simulink model "switched_load_R2021a"  (R2021a)
settings: Solver=VariableStepAuto  StartTime=0.0  StopTime=3  RelTol=1e-3
libraries: spsDiodeLib x15, spsSeriesRLCBranchLib x13, spsIGBTDiodeLib x12, spsVoltageMeasurementLib x6, spsCurrentMeasurementLib x6, simulink x2, spsIGBTLib x2, spsThreePhaseVIMeasurementLib x1, spsThreePhaseSourceLib x1, spsGroundLib x1, spspowerguiLib x1
settings Model: Creator=amogh  LastModifiedBy=amogh
settings DebuggingCC: UnconnectedInputMsg=none  UnconnectedOutputMsg=none  UnconnectedLineMsg=none
settings ModelReferenceCC: EnableRefExpFcnMdlSchedulingChecks=off
settings RTWCC: Description=Generic Real-Time Target  GPUComputeCapability=5.0  DLArmComputeVersion=20.02.1

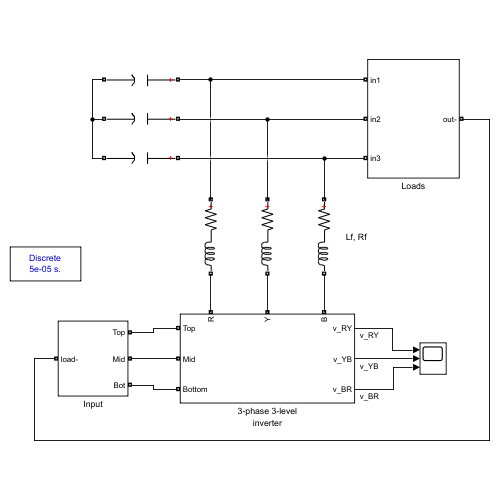
[thumbnail: Simulink's stored preview of the top-level diagram]
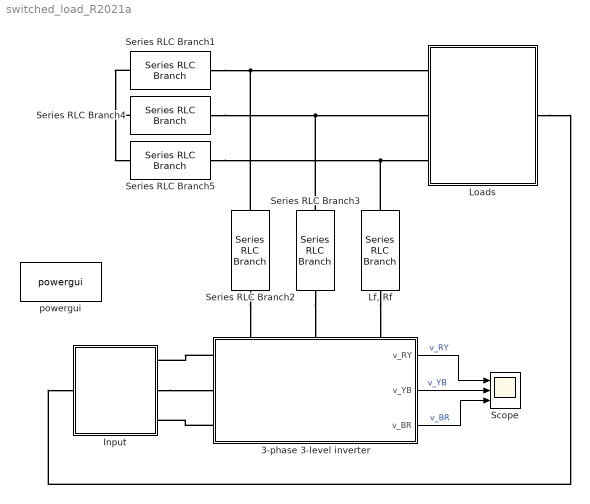
== system switched_load_R2021a ==
  3-phase 3-level inverter : Subsystem
      settings: PortSchema="{\"entries\":[{\"content\":{\"sides\":[{\"content\":{\"connectorIds\":[\"LConn1\",\"LConn2\",\"LConn3\"]},\"type\":\"ConnectorPlacement.EquallySpacedRectSide\",\"uuid\":\"13d4cf2c-4c1e-42a3-9432-c4e4ea2c8c55\"},{\"content\":{\"connectorIds\":[\"Out1\",\"Out2\",\"Out3\"],\"side\":\"RIGHT\"},\"type\":\"ConnectorPlacement.EquallySpacedRectSide\",\"uuid\":\"789192d8-f493-444e-b6ae-5a6372a819a0\"},{\"content\":{\"connectorIds\":[\"LConn4\",\"LConn5\",\"LConn6\"],\"side\":\"TOP\"},\"type\":\"ConnectorPlacement.EquallySpacedRectSide\",\"uuid\":\"d4a8605d-32e8-489f-b368-c8e22b15ad13\"}]},\"type\":\"ConnectorPlacement.EquallySpacedConnector\",\"uuid\":\"3af644a1-665b-410e-abe8-e1731342a0b4\"}],\"packageUris\":[\"http://schema.mathworks.com/mf0/Connector/R2020b\"],\"version\":\"1.0\"}"
  Input : Subsystem
  "Lf, Rf" : spsSeriesRLCBranchLib/Series RLC Branch  LConnTagsString=__new0  RConnTagsString=__new0  BranchType=RL  Resistance=0.01  Inductance=20e-3  SetiL0=off  InitialCurrent=0  Capacitance=1e-6  Setx0=off  InitialVoltage=0  Measurements=None
  Loads : Subsystem
  Scope : Scope  NumInputPorts=3
  Series RLC Branch1 : spsSeriesRLCBranchLib/Series RLC Branch  LConnTagsString=__new0  RConnTagsString=__new0  BranchType=C  Resistance=1  Inductance=20e-3  SetiL0=off  InitialCurrent=0  Capacitance=40e-6  Setx0=off  InitialVoltage=0  Measurements=None
  Series RLC Branch2 : spsSeriesRLCBranchLib/Series RLC Branch  LConnTagsString=__new0  RConnTagsString=__new0  BranchType=RL  Resistance=0.01  Inductance=20e-3  SetiL0=off  InitialCurrent=0  Capacitance=1e-6  Setx0=off  InitialVoltage=0  Measurements=None
  Series RLC Branch3 : spsSeriesRLCBranchLib/Series RLC Branch  LConnTagsString=__new0  RConnTagsString=__new0  BranchType=RL  Resistance=0.01  Inductance=20e-3  SetiL0=off  InitialCurrent=0  Capacitance=1e-6  Setx0=off  InitialVoltage=0  Measurements=None
  Series RLC Branch4 : spsSeriesRLCBranchLib/Series RLC Branch  LConnTagsString=__new0  RConnTagsString=__new0  BranchType=C  Resistance=1  Inductance=20e-3  SetiL0=off  InitialCurrent=0  Capacitance=40e-6  Setx0=off  InitialVoltage=0  Measurements=None
  Series RLC Branch5 : spsSeriesRLCBranchLib/Series RLC Branch  LConnTagsString=__new0  RConnTagsString=__new0  BranchType=C  Resistance=1  Inductance=20e-3  SetiL0=off  InitialCurrent=0  Capacitance=40e-6  Setx0=off  InitialVoltage=0  Measurements=None
  powergui : spspowerguiLib/powergui  Priority=1  SimulationMode=Discrete  SampleTime=50e-6  frequency=60  Iterations=50  frequencyindice=0  Pbase=100e6  ErrMax=1e-4  UnitsV=kV  UnitsW=MW  buscounter=0  FunctionMessages=off  echomessages=off  EnableUseOfTLC=off  CurrentSourceSwitches=off  DisableSnubberDevices=off  DisableRonSwitches=off  DisableVfSwitches=off  DisplayEquations=off  AutomaticDiscreteSolvers=off  SolverType=Tustin/Backward Euler (TBE)  Interpol=off  ExternalGateDelay=off  methode=off  Ts=100  x0status=blocks  SPID=on  SwTol=0  HookPort=off  NonlinearTolerance=1e-4  nMaxIteration=100  ContinueOnMaxIteration=off  RestoreLinks=warning  ResistiveCurrentMeasurement=off  Frange=[0:2:500]  Ylog=off  Xlog=on  ShowGrid=off  save=off  variable=ZData  structure=0  ZoomFFT=off  StartTime=0.0  cycles=1  DisplayStyle=1  fundamental=60  FreqAxis=off  MaxFrequency=1000  frequencyindicesteady=1  RmsSteady=1  display=off
  wires:
  3-phase 3-level inverter/3(v_BR) -> Scope/3  "v_BR"
  3-phase 3-level inverter/2(v_YB) -> Scope/2  "v_YB"
  3-phase 3-level inverter/1(v_RY) -> Scope/1  "v_RY"
  connections:
  Series RLC Branch1/LConn1 -- Loads/LConn1 -- Series RLC Branch2/LConn1
  Series RLC Branch5/LConn1 -- Loads/LConn3 -- "Lf, Rf"/LConn1
  Series RLC Branch4/RConn1 -- Series RLC Branch5/RConn1 -- Series RLC Branch1/RConn1
  Series RLC Branch4/LConn1 -- Loads/LConn2 -- Series RLC Branch3/LConn1
  3-phase 3-level inverter/LConn3 -- Input/RConn3
  Input/RConn2 -- 3-phase 3-level inverter/LConn2
  3-phase 3-level inverter/LConn1 -- Input/RConn1
  Series RLC Branch2/RConn1 -- 3-phase 3-level inverter/LConn4
  Series RLC Branch3/RConn1 -- 3-phase 3-level inverter/LConn5
  "Lf, Rf"/RConn1 -- 3-phase 3-level inverter/LConn6
  Loads/RConn1 -- Input/LConn1

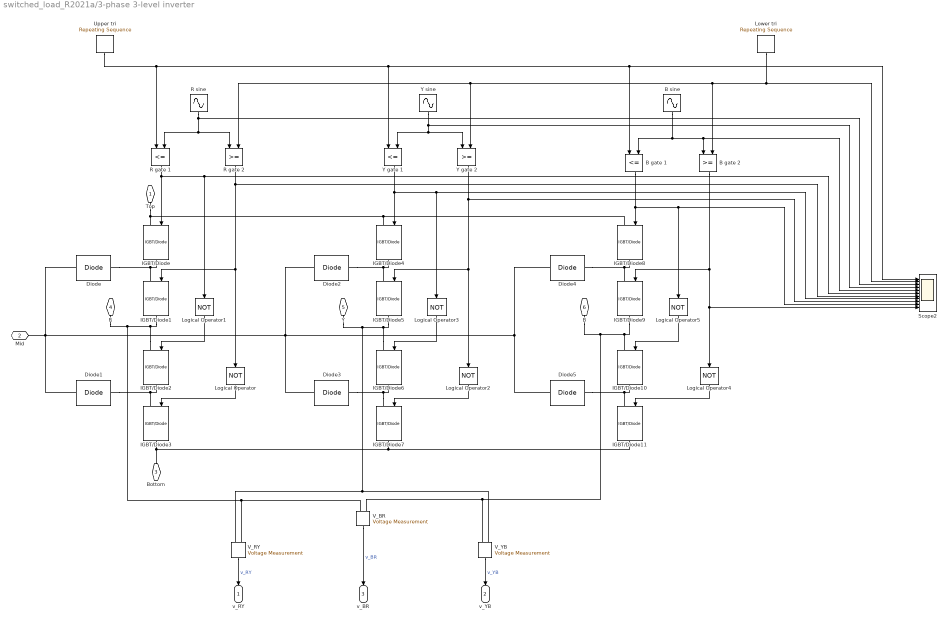
== system switched_load_R2021a/3-phase 3-level inverter ==
  B gate 1 : RelationalOperator  Operator=<=  OutDataTypeStr=boolean  RndMeth=Simplest
  B gate 2 : RelationalOperator  OutDataTypeStr=boolean  RndMeth=Simplest
  B sine : Sin  Frequency=100*pi  Phase=2*pi/3  SampleTime=0
  Diode{,1..5} (6 alike) : spsDiodeLib/Diode  Ron=0.001  Lon=0  Vf=0  IC=0  UseSnubber=0  Rs=500  Cs=250e-9  Measurements=off
  IGBT/Diode{,1..11} (12 alike) : spsIGBTDiodeLib/IGBT//Diode  Ron=1e-3  Rs=1e5  Cs=inf  Measurements=off
  Logical Operator{,1..5} (6 alike) : Logic  Operator=NOT  AllPortsSameDT=off  OutDataTypeStr=boolean
  Lower tri : simulink/Sources/Repeating Sequence  rep_seq_t=[0 0.0002 0.0004 0.0006 0.0008]  rep_seq_y=[-0.5 -1 -0.5 0 -0.5]
  R gate 1 : RelationalOperator  Operator=<=  OutDataTypeStr=boolean  RndMeth=Simplest
  R gate 2 : RelationalOperator  OutDataTypeStr=boolean  RndMeth=Simplest
  R sine : Sin  Frequency=100*pi  SampleTime=0
  Scope2 : Scope  NumInputPorts=11
  Upper tri : simulink/Sources/Repeating Sequence  rep_seq_t=[0 0.0002 0.0004 0.0006 0.0008]  rep_seq_y=[0.5 0 0.5 1 0.5]
  V_BR : spsVoltageMeasurementLib/Voltage Measurement  PhasorSimulation=off  OutputType=Complex  PSBequivalent=0
  V_RY : spsVoltageMeasurementLib/Voltage Measurement  PhasorSimulation=off  OutputType=Complex  PSBequivalent=0
  V_YB : spsVoltageMeasurementLib/Voltage Measurement  PhasorSimulation=off  OutputType=Complex  PSBequivalent=0
  Y gate 1 : RelationalOperator  Operator=<=  OutDataTypeStr=boolean  RndMeth=Simplest
  Y gate 2 : RelationalOperator  OutDataTypeStr=boolean  RndMeth=Simplest
  Y sine : Sin  Frequency=100*pi  Phase=-2*pi/3  SampleTime=0
  Top : PMIOPort  Side=Left
  Mid : PMIOPort  Port=2  Side=Left
  Bottom : PMIOPort  Port=3  Side=Left
  R : PMIOPort  Port=4  Side=Left
  Y : PMIOPort  Port=5  Side=Left
  B : PMIOPort  Port=6  Side=Left
  v_RY : Outport
  v_YB : Outport  Port=2
  v_BR : Outport  Port=3
  wires:
  Logical Operator/1 -> IGBT/Diode3/1
  R gate 1/1 -> IGBT/Diode/1, Logical Operator1/1, Scope2/6
  B sine/1 -> Scope2/5, B gate 2/1, B gate 1/2
  Y gate 1/1 -> IGBT/Diode4/1, Logical Operator3/1, Scope2/8
  Lower tri/1 -> B gate 2/2, Y gate 2/2, R gate 2/2, Scope2/2
  Y gate 2/1 -> IGBT/Diode5/1, Logical Operator2/1, Scope2/9
  R gate 2/1 -> Logical Operator/1, IGBT/Diode1/1, Scope2/7
  Logical Operator2/1 -> IGBT/Diode7/1
  Upper tri/1 -> Y gate 1/1, B gate 1/1, Scope2/1, R gate 1/1
  Y sine/1 -> Y gate 2/1, Y gate 1/2, Scope2/4
  B gate 1/1 -> IGBT/Diode8/1, Scope2/10, Logical Operator5/1
  R sine/1 -> R gate 2/1, R gate 1/2, Scope2/3
  B gate 2/1 -> Scope2/11, Logical Operator4/1, IGBT/Diode9/1
  V_BR/1 -> v_BR/1  "v_BR"
  Logical Operator3/1 -> IGBT/Diode6/1
  Logical Operator5/1 -> IGBT/Diode10/1
  Logical Operator4/1 -> IGBT/Diode11/1
  Logical Operator1/1 -> IGBT/Diode2/1
  V_YB/1 -> v_YB/1  "v_YB"
  V_RY/1 -> v_RY/1  "v_RY"
  connections:
  IGBT/Diode7/RConn1 -- Bottom/RConn1 -- IGBT/Diode3/RConn1 -- IGBT/Diode11/RConn1
  Diode/RConn1 -- IGBT/Diode1/LConn1 -- IGBT/Diode/RConn1
  IGBT/Diode2/LConn1 -- R/RConn1 -- V_RY/LConn1 -- V_BR/LConn2 -- IGBT/Diode1/RConn1
  Diode2/RConn1 -- IGBT/Diode5/LConn1 -- IGBT/Diode4/RConn1
  IGBT/Diode6/LConn1 -- Y/RConn1 -- V_YB/LConn1 -- V_RY/LConn2 -- IGBT/Diode5/RConn1
  IGBT/Diode/LConn1 -- Top/RConn1 -- IGBT/Diode8/LConn1 -- IGBT/Diode4/LConn1
  Diode1/LConn1 -- IGBT/Diode2/RConn1 -- IGBT/Diode3/LConn1
  V_YB/LConn2 -- IGBT/Diode9/RConn1 -- IGBT/Diode10/LConn1 -- B/RConn1 -- V_BR/LConn1
  Diode4/RConn1 -- IGBT/Diode9/LConn1 -- IGBT/Diode8/RConn1
  Diode5/RConn1 -- Mid/RConn1 -- Diode/LConn1 -- Diode1/RConn1 -- Diode2/LConn1 -- Diode3/RConn1 -- Diode4/LConn1
  IGBT/Diode7/LConn1 -- IGBT/Diode6/RConn1 -- Diode3/LConn1
  Diode5/LConn1 -- IGBT/Diode10/RConn1 -- IGBT/Diode11/LConn1

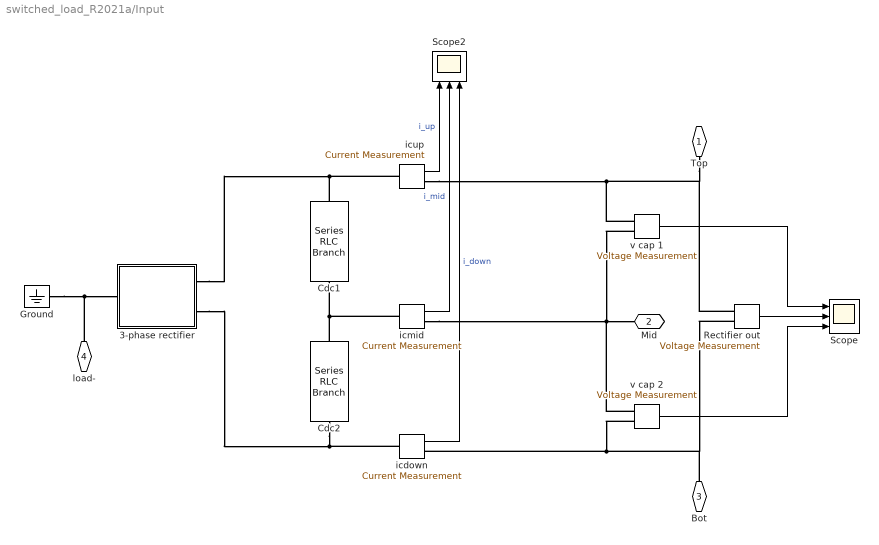
== system switched_load_R2021a/Input ==
  3-phase rectifier : Subsystem
  Cdc1 : spsSeriesRLCBranchLib/Series RLC Branch  LConnTagsString=__new0  RConnTagsString=__new0  BranchType=C  Resistance=1  Inductance=1e-3  SetiL0=off  InitialCurrent=0  Capacitance=500e-6  Setx0=off  InitialVoltage=0  Measurements=None
  Cdc2 : spsSeriesRLCBranchLib/Series RLC Branch  LConnTagsString=__new0  RConnTagsString=__new0  BranchType=C  Resistance=1  Inductance=1e-3  SetiL0=off  InitialCurrent=0  Capacitance=500e-6  Setx0=off  InitialVoltage=0  Measurements=None
  Ground : spsGroundLib/Ground  LConnTagsString=a
  Rectifier out : spsVoltageMeasurementLib/Voltage Measurement  PhasorSimulation=off  OutputType=Complex  PSBequivalent=0
  Scope : Scope  NumInputPorts=3
  Scope2 : Scope  NumInputPorts=3
  icdown : spsCurrentMeasurementLib/Current Measurement  PhasorSimulation=off  OutputType=Complex  PSBequivalent=0
  icmid : spsCurrentMeasurementLib/Current Measurement  PhasorSimulation=off  OutputType=Complex  PSBequivalent=0
  icup : spsCurrentMeasurementLib/Current Measurement  PhasorSimulation=off  OutputType=Complex  PSBequivalent=0
  v cap 1 : spsVoltageMeasurementLib/Voltage Measurement  PhasorSimulation=off  OutputType=Complex  PSBequivalent=0
  v cap 2 : spsVoltageMeasurementLib/Voltage Measurement  PhasorSimulation=off  OutputType=Complex  PSBequivalent=0
  Top : PMIOPort  Side=Right
  Mid : PMIOPort  Port=2  Side=Right
  Bot : PMIOPort  Port=3  Side=Right
  load- : PMIOPort  Port=4  Side=Left
  wires:
  icmid/1 -> Scope2/2  "i_mid"
  icdown/1 -> Scope2/3  "i_down"
  icup/1 -> Scope2/1  "i_up"
  Rectifier out/1 -> Scope/2
  v cap 1/1 -> Scope/1
  v cap 2/1 -> Scope/3
  connections:
  Ground/LConn1 -- 3-phase rectifier/LConn1 -- load-/RConn1
  icmid/LConn1 -- Cdc2/LConn1 -- Cdc1/RConn1
  v cap 2/LConn2 -- icdown/RConn1 -- Bot/RConn1 -- Rectifier out/LConn2
  Cdc2/RConn1 -- icdown/LConn1 -- 3-phase rectifier/RConn2
  Cdc1/LConn1 -- 3-phase rectifier/RConn1 -- icup/LConn1
  icup/RConn1 -- Rectifier out/LConn1 -- Top/RConn1 -- v cap 1/LConn1
  v cap 2/LConn1 -- v cap 1/LConn2 -- icmid/RConn1 -- Mid/RConn1

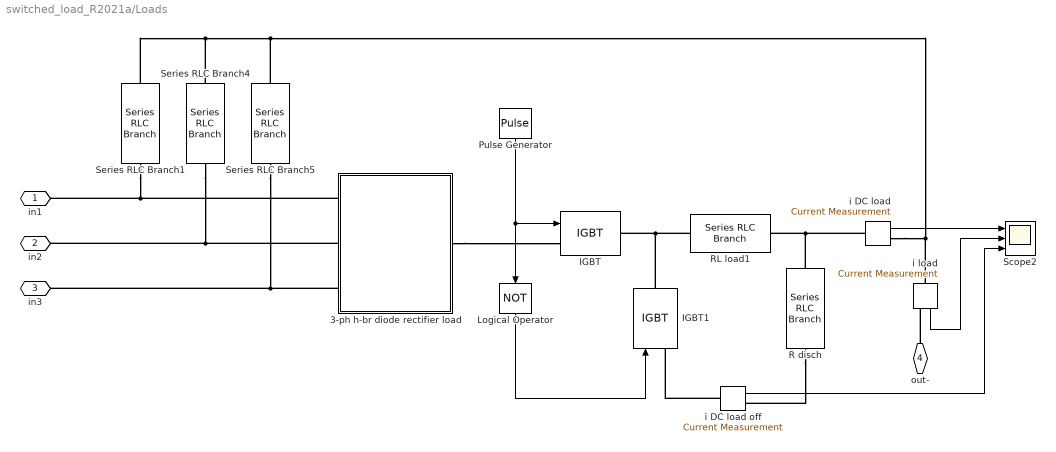
== system switched_load_R2021a/Loads ==
  3-ph h-br diode rectifier load : Subsystem
  IGBT : spsIGBTLib/IGBT  Ron=0.001  Lon=0  Vf=1  Tf=1e-6  Tt=2e-6  IC=0  Rs=1e5  Cs=inf  Measurements=off
  IGBT1 : spsIGBTLib/IGBT  Ron=0.001  Lon=0  Vf=1  Tf=1e-6  Tt=2e-6  IC=0  Rs=1e5  Cs=inf  Measurements=off
  Logical Operator : Logic  Operator=NOT  AllPortsSameDT=off  OutDataTypeStr=boolean
  Pulse Generator : DiscretePulseGenerator  PulseType=Time based  PulseWidth=50
  R disch : spsSeriesRLCBranchLib/Series RLC Branch  LConnTagsString=__new0  RConnTagsString=__new0  BranchType=R  Resistance=1  Inductance=0.1  SetiL0=off  InitialCurrent=0  Capacitance=1e-6  Setx0=off  InitialVoltage=0  Measurements=None
  RL load1 : spsSeriesRLCBranchLib/Series RLC Branch  LConnTagsString=__new0  RConnTagsString=__new0  BranchType=RL  Resistance=0.1  Inductance=0.1  SetiL0=off  InitialCurrent=0  Capacitance=1e-6  Setx0=off  InitialVoltage=0  Measurements=None
  Scope2 : Scope  NumInputPorts=3
  Series RLC Branch1 : spsSeriesRLCBranchLib/Series RLC Branch  LConnTagsString=__new0  RConnTagsString=__new0  BranchType=RL  Resistance=3e1  Inductance=2e-2  SetiL0=off  InitialCurrent=0  Capacitance=1e-6  Setx0=off  InitialVoltage=0  Measurements=None
  Series RLC Branch4 : spsSeriesRLCBranchLib/Series RLC Branch  LConnTagsString=__new0  RConnTagsString=__new0  BranchType=RL  Resistance=6e1  Inductance=3e-2  SetiL0=off  InitialCurrent=0  Capacitance=1e-6  Setx0=off  InitialVoltage=0  Measurements=None
  Series RLC Branch5 : spsSeriesRLCBranchLib/Series RLC Branch  LConnTagsString=__new0  RConnTagsString=__new0  BranchType=RL  Resistance=9e1  Inductance=4e-2  SetiL0=off  InitialCurrent=0  Capacitance=1e-6  Setx0=off  InitialVoltage=0  Measurements=None
  i DC load : spsCurrentMeasurementLib/Current Measurement  PhasorSimulation=off  OutputType=Complex  PSBequivalent=0
  i DC load off : spsCurrentMeasurementLib/Current Measurement  PhasorSimulation=off  OutputType=Complex  PSBequivalent=0
  i load : spsCurrentMeasurementLib/Current Measurement  PhasorSimulation=off  OutputType=Complex  PSBequivalent=0
  in1 : PMIOPort  Side=Left
  in2 : PMIOPort  Port=2  Side=Left
  in3 : PMIOPort  Port=3  Side=Left
  out- : PMIOPort  Port=4  Side=Right
  wires:
  i DC load/1 -> Scope2/1
  i load/1 -> Scope2/2
  i DC load off/1 -> Scope2/3
  Pulse Generator/1 -> IGBT/1, Logical Operator/1
  Logical Operator/1 -> IGBT1/1
  connections:
  Series RLC Branch4/LConn1 -- Series RLC Branch1/LConn1 -- Series RLC Branch5/LConn1 -- i load/LConn1 -- i DC load/RConn1
  Series RLC Branch1/RConn1 -- 3-ph h-br diode rectifier load/LConn1 -- in1/RConn1
  3-ph h-br diode rectifier load/LConn3 -- Series RLC Branch5/RConn1 -- in3/RConn1
  Series RLC Branch4/RConn1 -- 3-ph h-br diode rectifier load/LConn2 -- in2/RConn1
  i DC load/LConn1 -- R disch/RConn1 -- RL load1/LConn1
  out-/RConn1 -- i load/RConn1
  3-ph h-br diode rectifier load/RConn1 -- IGBT/LConn1
  RL load1/RConn1 -- IGBT1/RConn1 -- IGBT/RConn1
  i DC load off/LConn1 -- IGBT1/LConn1
  R disch/LConn1 -- i DC load off/RConn1

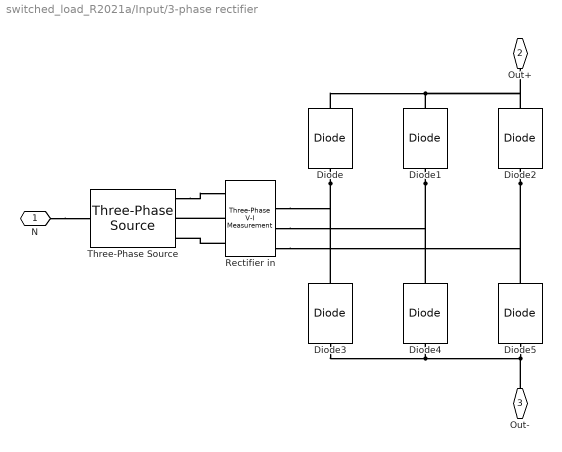
== system switched_load_R2021a/Input/3-phase rectifier ==
  Diode{,1..5} (6 alike) : spsDiodeLib/Diode  Ron=0.001  Lon=0  Vf=0  IC=0  UseSnubber=0  Rs=500  Cs=250e-9  Measurements=off
  Rectifier in : spsThreePhaseVIMeasurementLib/Three-Phase V-I Measurement  VoltageMeasurement=phase-to-ground  SetLabelV=off  LabelV=Vabc  Vpu=off  VpuLL=off  CurrentMeasurement=no  SetLabelI=off  LabelI=Iabc  Ipu=off  Pbase=100e6  Vbase=500e3  OutputType=Complex  PhasorSimulation=off  PSBequivalent=0
  Three-Phase Source : spsThreePhaseSourceLib/Three-Phase Source  InternalConnection=Yn  VoltagePhases=off  Voltage=230*sqrt(3)  PhaseAngle=0  Voltage_phases=[25e3 25e3 25e3]/sqrt(3)  PhaseAngles_phases=[0 -120 +120]  Frequency=50  NonIdealSource=off  SpecifyImpedance=off  Resistance=0.8929  Inductance=16.58e-3  ShortCircuitLevel=100e6  BaseVoltage=25e3  XRratio=7  BusType=swing  Pref=10e3  Qref=0  Prefabc=[10e3, 10e3, 10e3]  Qrefabc=[0, 0, 0]  Qmin=-inf  Qmax=inf
  N : PMIOPort  Side=Left
  Out+ : PMIOPort  Port=2  Side=Right
  Out- : PMIOPort  Port=3  Side=Right
  connections:
  Diode1/LConn1 -- Diode4/RConn1 -- Rectifier in/RConn2
  Diode2/LConn1 -- Diode5/RConn1 -- Rectifier in/RConn3
  Diode/LConn1 -- Diode3/RConn1 -- Rectifier in/RConn1
  Three-Phase Source/RConn1 -- Rectifier in/LConn1
  Rectifier in/LConn2 -- Three-Phase Source/RConn2
  Rectifier in/LConn3 -- Three-Phase Source/RConn3
  Diode/RConn1 -- Diode2/RConn1 -- Out+/RConn1 -- Diode1/RConn1
  N/RConn1 -- Three-Phase Source/LConn1
  Diode3/LConn1 -- Diode5/LConn1 -- Out-/RConn1 -- Diode4/LConn1

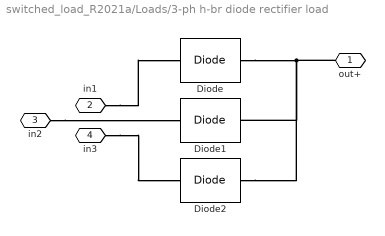
== system switched_load_R2021a/Loads/3-ph h-br diode rectifier load ==
  Diode : spsDiodeLib/Diode  Ron=0.001  Lon=0  Vf=0  IC=0  UseSnubber=0  Rs=500  Cs=250e-9  Measurements=off
  Diode1 : spsDiodeLib/Diode  Ron=0.001  Lon=0  Vf=0  IC=0  UseSnubber=0  Rs=500  Cs=250e-9  Measurements=off
  Diode2 : spsDiodeLib/Diode  Ron=0.001  Lon=0  Vf=0  IC=0  UseSnubber=0  Rs=500  Cs=250e-9  Measurements=off
  out+ : PMIOPort  Side=Right
  in1 : PMIOPort  Port=2  Side=Left
  in2 : PMIOPort  Port=3  Side=Left
  in3 : PMIOPort  Port=4  Side=Left
  connections:
  in1/RConn1 -- Diode/LConn1
  Diode/RConn1 -- out+/RConn1 -- Diode2/RConn1 -- Diode1/RConn1
  in2/RConn1 -- Diode1/LConn1
  in3/RConn1 -- Diode2/LConn1
